simulink model "Conveyer_Belt_System"  (R2023a)
settings: Solver=VariableStepAuto  StartTime=0.0  StopTime=50  RelTol=1e-3
values from neighbouring files (symbols this model uses):
  Kb = 23e-3    (= 0.023)    [UpgradedConveyorBeltParameters.m]
  Kt = 23e-3    (= 0.023)    [UpgradedConveyorBeltParameters.m]
  L = 0.1    [UpgradedConveyorBeltParameters.m]
  R = 0.71    [UpgradedConveyorBeltParameters.m]
undefined symbols (not defined in the file or in its folder): J, Kd
libraries: SignalEditorBlockLib x4, slpidlib x1
settings Model: Creator=M3tal  LastModifiedBy=M3tal
settings ConfigComp: PLC_TargetIDE=generic  PLC_MultiTBSigbuilderTimeRange=off  PLC_FoldFBCallOutputVar=off  PLC_RemoveUnusedSSMethodCallArguments=off  PLC_UseCallOutputArgSyntax=off  PLC_EnableUnsignedAndDoubleTypes=off  PLC_EnableUDTSplitting=off  PLC_MaxFieldsInUDT=500  PLC_InlineEnumCastFunction=off

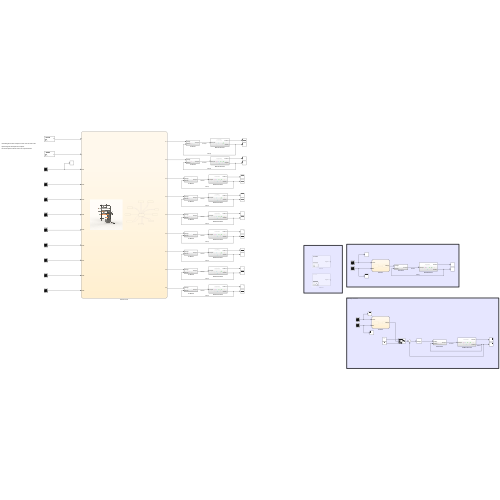
[thumbnail: Simulink's stored preview of the top-level diagram]
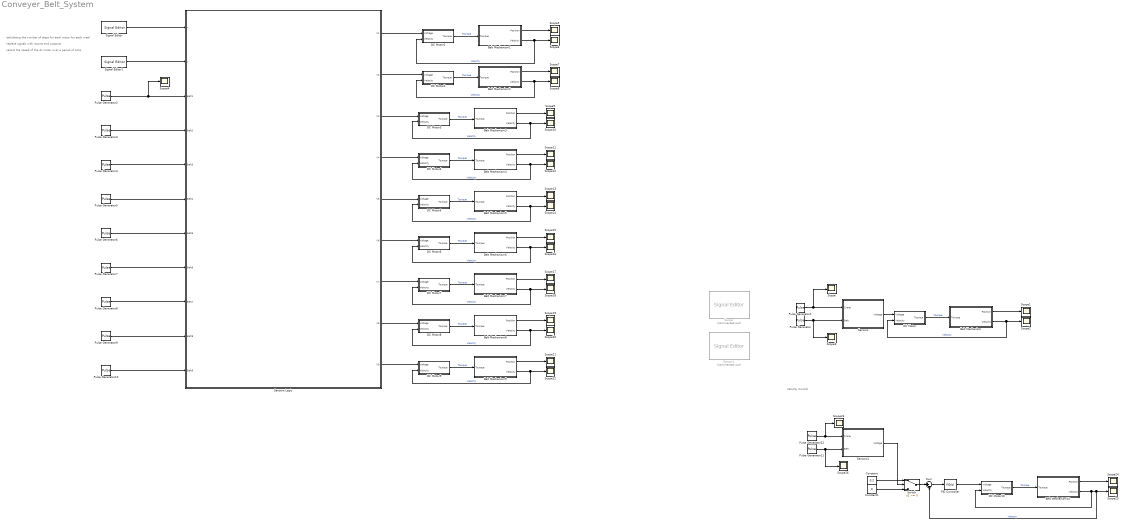
== system Conveyer_Belt_System ==
  note: -record the speed of the dc motor over a period of time
  note: -replace signals with inports and outports
  note: -caluclating the number of steps for each motor for each meal
  note: Velocity Control
  Belt Mechanism : Subsystem
  Belt Mechanism1 : Subsystem
  Belt Mechanism10 : Subsystem
  Belt Mechanism2 : Subsystem
  Belt Mechanism3 : Subsystem
  Belt Mechanism4 : Subsystem
  Belt Mechanism5 : Subsystem
  Belt Mechanism6 : Subsystem
  Belt Mechanism7 : Subsystem
  Belt Mechanism8 : Subsystem
  Belt Mechanism9 : Subsystem
  Constant : Constant  Value=0.2
  Constant1 : Constant  Value=0
  DC Motor : Subsystem
  DC Motor1 : Subsystem
  DC Motor10 : Subsystem
  DC Motor2 : Subsystem
  DC Motor3 : Subsystem
  DC Motor4 : Subsystem
  DC Motor5 : Subsystem
  DC Motor6 : Subsystem
  DC Motor7 : Subsystem
  DC Motor8 : Subsystem
  DC Motor9 : Subsystem
  PID Controller : slpidlib/PID Controller  Controller=PID  Form=Parallel  TimeDomain=Continuous-time  UseExternalTs=off  SampleTime=-1  IntegratorMethod=Forward Euler  FilterMethod=Forward Euler  ControllerParametersSource=internal  P=62.3819569355445  I=32.9771532942244  UseKiTs=off  D=11.2137291947193  N=1.39512955862012  UseFilter=on  TunerSelectOption=Transfer Function Based (PID Tuner App)  InitialConditionSource=internal  InitialConditionForIntegrator=0  InitialConditionForFilter=0  DifferentiatorICPrevScaledInput=0  ExternalReset=none  TrackingMode=off  Kt=1  LimitOutput=off  SatLimitsSource=internal  UpperSaturationLimit=inf  LowerSaturationLimit=-inf  LinearizeAsGain=on  AntiWindupMode=none  Kb=1  LimitIntegrator=off  UpperIntegratorSaturationLimit=inf  LowerIntegratorSaturationLimit=-inf  POutMin=[]  POutMax=[]  IOutMin=[]  IOutMax=[]  DOutMin=[]  DOutMax=[]  NOutMin=[]  NOutMax=[]  SumOutMin=[]  SumOutMax=[]  SaturationOutMin=[]  SaturationOutMax=[]  PParamMin=[]  PParamMax=[]  IParamMin=[]  IParamMax=[]  DParamMin=[]  DParamMax=[]  NParamMin=[]  NParamMax=[]  KbParamMin=[]  KbParamMax=[]  KtParamMin=[]  KtParamMax=[]  KbOutMin=[]  KbOutMax=[]  KtOutMin=[]  KtOutMax=[]  IntegratorOutMin=[]  IntegratorOutMax=[]  FilterOutMin=[]  FilterOutMax=[]  SumI1OutMin=[]  SumI1OutMax=[]  SumI2OutMin=[]  SumI2OutMax=[]  SumI3OutMin=[]  SumI3OutMax=[]  SumI4OutMin=[]  SumI4OutMax=[]  SumDOutMin=[]  SumDOutMax=[]  DifferentiatorOutMin=[]  DifferentiatorOutMax=[]  FilterDiffOutCoefMin=[]  FilterDiffOutCoefMax=[]  ReciprocalOutMin=[]  ReciprocalOutMax=[]  SumDenOutMin=[]  SumDenOutMax=[]  SumNumOutMin=[]  SumNumOutMax=[]  DivideOutMin=[]  DivideOutMax=[]  UdiffTsProdOutMin=[]  UdiffTsProdOutMax=[]  NTsProdOutMin=[]  NTsProdOutMax=[]  UintegralTsProdOutMin=[]  UintegralTsProdOutMax=[]  UngainTsProdOutMin=[]  UngainTsProdOutMax=[]  ClampingZeroOutDataTypeStr=Inherit: Inherit via back propagation  ClampingZeroOutMin=[]  ClampingZeroOutMax=[]  FilterDenConstantOutDataTypeStr=Inherit: Inherit via back propagation  FilterDenConstantOutMin=[]  FilterDenConstantOutMax=[]  PCopyOutDataTypeStr=Inherit: Inherit via back propagation  PCopyOutMin=[]  PCopyOutMax=[]  NCopyOutDataTypeStr=Inherit: Inherit via back propagation  NCopyOutMin=[]  NCopyOutMax=[]  IntegratorContinuousStateAttributes=''  IntegratorStateMustResolveToSignalObject=off  IntegratorRTWStateStorageClass=Auto  FilterContinuousStateAttributes=''  FilterStateMustResolveToSignalObject=off  FilterRTWStateStorageClass=Auto  ParallelPVariant=InternalParameters  IdealPVariant=Disabled  IVariant=InternalParameters  DVariant=InternalParameters  IntegratorVariant=Continuous  SatVariant=Disabled  AWVariant=Passthrough  PCopyVariant=Disabled  TRVariant=Disabled  FdbkBlocksVariant=Forward  IdealPFdbkVariant=Disabled  SatFdbkVariant=Disabled  DerivativeFilterVariant=ContFilter  NVariant=InternalParameters  NCopyVariant=Disabled  FilterICVariant=InternalICsFilter  IntegratorICVariant=InternalICs  ExternalResetVariant=Disabled  TRSumVariant=Passthrough  SumFdbkVariant=Disabled  SumVariant=Sum_PID  TsampFilterVariant=InternalTs  TsampNgainVariant=Passthrough  TsampIntegralVariant=Disabled_SignalSpec  ExternalSaturationOutDataTypeStr=Inherit: Same as second input
  Pulse Generator : DiscretePulseGenerator  PulseType=Time based  Period=40  PhaseDelay=20
  Pulse Generator1 : DiscretePulseGenerator  PulseType=Time based  Period=50  PhaseDelay=5
  Pulse Generator{3..10} (8 alike) : DiscretePulseGenerator  PulseType=Time based  Amplitude=0  Period=50  PhaseDelay=5
  Pulse Generator11 : DiscretePulseGenerator  PulseType=Time based  Period=40  PhaseDelay=20
  Pulse Generator12 : DiscretePulseGenerator  PulseType=Time based  Period=50  PhaseDelay=5
  Pulse Generator2 : DiscretePulseGenerator  PulseType=Time based  Period=50  PulseWidth=50  PhaseDelay=25
  Scope{,1..26} (27 alike) : Scope
  Sensor : SignalEditorBlockLib/Signal Editor  Commented=on  FileName=Crane_Sensor.mat  ActiveScenario=Scenario  ActiveSignal=Crane signal  IsBus=off  OutputBusObjectStr=Bus: BusObject  SampleTime=0  Interpolate=off  ZeroCross=off  OutputAfterFinalValue=Setting to zero  Unit=inherit  PreserveSignalName=on  ApplySigPropsToAllScenarios=on
  Sensor1 : SignalEditorBlockLib/Signal Editor  Commented=on  FileName=Belt_Sensor.mat  ActiveScenario=Scenario  ActiveSignal=Belt Signal  IsBus=off  OutputBusObjectStr=Bus: BusObject  SampleTime=0  Interpolate=off  ZeroCross=off  OutputAfterFinalValue=Setting to zero  Unit=inherit  PreserveSignalName=on  ApplySigPropsToAllScenarios=on
  Sensors : Stateflow chart  TreatAsAtomicUnit=on
  Sensors Logic : Stateflow chart  TreatAsAtomicUnit=on
      settings: PortSchema="{\"entries\":[{\"content\":{\"sides\":[{\"content\":{\"connectorIds\":[\"In10\",\"In11\",\"In1\",\"In2\",\"In3\",\"In4\",\"In5\",\"In6\",\"In7\",\"In8\",\"In9\"]},\"type\":\"ConnectorPlacement.EquallySpacedRectSide\",\"uuid\":\"dd9ce701-3689-4654-9b21-5529dab0541a\"},{\"content\":{\"connectorIds\":[\"Out1\",\"Out2\",\"Out3\",\"Out4\",\"Out5\",\"Out6\",\"Out7\",\"Out8\",\"Out9\"],\"side\":\"RIGHT\"},\"type\":\"ConnectorPlacement.EquallySpacedRectSide\",\"uuid\":\"ff8f0f67-846c-4703-aeda-d87216d47c92\"},{\"content\":{\"side\":\"TOP\"},\"type\":\"ConnectorPlacement.EquallySpacedRectSide\",\"uuid\":\"ae968bb7-da0f-44fd-802b-06f57922bbce\"}]},\"type\":\"ConnectorPlacement.EquallySpacedConnector\",\"uuid\":\"820653e5-881f-4b8b-9810-894dc5dde637\"}],\"packageUris\":[\"http://schema.mathworks.com/mf0/Connector/R2020b\"],\"version\":\"1.0\"}"
  Sensors1 : Stateflow chart  TreatAsAtomicUnit=on
  Signal Editor : SignalEditorBlockLib/Signal Editor  FileName=X_Position.mat  ActiveScenario=Scenario  ActiveSignal=X  IsBus=off  OutputBusObjectStr=Bus: BusObject  SampleTime=0  Interpolate=off  ZeroCross=off  OutputAfterFinalValue=Setting to zero  Unit=inherit  PreserveSignalName=on  ApplySigPropsToAllScenarios=on
  Signal Editor1 : SignalEditorBlockLib/Signal Editor  FileName=Y_Position.mat  ActiveScenario=Scenario  ActiveSignal=Y  IsBus=off  OutputBusObjectStr=Bus: BusObject  SampleTime=0  Interpolate=off  ZeroCross=off  OutputAfterFinalValue=Setting to zero  Unit=inherit  PreserveSignalName=on  ApplySigPropsToAllScenarios=on
  Sum : Sum  Inputs=|+-
  Switch : Switch  Criteria=u2 ~= 0  Threshold=1  SaturateOnIntegerOverflow=off  InputSameDT=off
  wires:
  Belt Mechanism/1(Position) -> Scope1/1
  DC Motor/1(Tourque) -> Belt Mechanism/1(Tourque)  "Tourque"
  Belt Mechanism/2(Velocity) -> Scope2/1, DC Motor/2(Velocity)  "Velocity"
  Pulse Generator/1 -> Scope3/1, Sensors/2(Belt)
  Pulse Generator1/1 -> Scope/1, Sensors/1(Crane)
  Pulse Generator2/1 -> Scope4/1, Sensors Logic/1(Belt1)
  Pulse Generator3/1 -> Sensors Logic/2(Belt2)
  Pulse Generator4/1 -> Sensors Logic/3(Belt3)
  Pulse Generator5/1 -> Sensors Logic/4(Belt4)
  Pulse Generator6/1 -> Sensors Logic/5(Belt5)
  Pulse Generator7/1 -> Sensors Logic/6(Belt6)
  Pulse Generator8/1 -> Sensors Logic/7(Belt7)
  Pulse Generator9/1 -> Sensors Logic/8(Belt8)
  Pulse Generator10/1 -> Sensors Logic/9(Belt9)
  Signal Editor1/1 -> Sensors Logic/11(y)
  Signal Editor/1 -> Sensors Logic/10(x)
  Belt Mechanism1/2(Velocity) -> Scope6/1, DC Motor1/2(Velocity)  "Velocity"
  DC Motor1/1(Tourque) -> Belt Mechanism1/1(Tourque)  "Tourque"
  Belt Mechanism1/1(Position) -> Scope5/1
  Belt Mechanism2/1(Position) -> Scope7/1
  DC Motor2/1(Tourque) -> Belt Mechanism2/1(Tourque)  "Tourque"
  Belt Mechanism2/2(Velocity) -> Scope8/1, DC Motor2/2(Velocity)  "Velocity"
  Belt Mechanism3/1(Position) -> Scope9/1
  DC Motor3/1(Tourque) -> Belt Mechanism3/1(Tourque)  "Tourque"
  Belt Mechanism3/2(Velocity) -> Scope10/1, DC Motor3/2(Velocity)  "Velocity"
  Belt Mechanism4/1(Position) -> Scope11/1
  DC Motor4/1(Tourque) -> Belt Mechanism4/1(Tourque)  "Tourque"
  Belt Mechanism4/2(Velocity) -> Scope12/1, DC Motor4/2(Velocity)  "Velocity"
  Belt Mechanism5/1(Position) -> Scope13/1
  DC Motor5/1(Tourque) -> Belt Mechanism5/1(Tourque)  "Tourque"
  Belt Mechanism5/2(Velocity) -> Scope14/1, DC Motor5/2(Velocity)  "Velocity"
  Belt Mechanism6/1(Position) -> Scope15/1
  DC Motor6/1(Tourque) -> Belt Mechanism6/1(Tourque)  "Tourque"
  Belt Mechanism6/2(Velocity) -> Scope16/1, DC Motor6/2(Velocity)  "Velocity"
  Belt Mechanism7/1(Position) -> Scope17/1
  DC Motor7/1(Tourque) -> Belt Mechanism7/1(Tourque)  "Tourque"
  Belt Mechanism7/2(Velocity) -> Scope18/1, DC Motor7/2(Velocity)  "Velocity"
  Belt Mechanism8/1(Position) -> Scope19/1
  DC Motor8/1(Tourque) -> Belt Mechanism8/1(Tourque)  "Tourque"
  Belt Mechanism8/2(Velocity) -> Scope20/1, DC Motor8/2(Velocity)  "Velocity"
  Belt Mechanism9/1(Position) -> Scope21/1
  DC Motor9/1(Tourque) -> Belt Mechanism9/1(Tourque)  "Tourque"
  Belt Mechanism9/2(Velocity) -> Scope22/1, DC Motor9/2(Velocity)  "Velocity"
  Sensors Logic/1(V1) -> DC Motor1/1(Voltage)
  Sensors Logic/2(V2) -> DC Motor2/1(Voltage)
  Sensors Logic/3(V3) -> DC Motor3/1(Voltage)
  Sensors Logic/4(V4) -> DC Motor4/1(Voltage)
  Sensors Logic/5(V5) -> DC Motor5/1(Voltage)
  Sensors Logic/6(V6) -> DC Motor6/1(Voltage)
  Sensors Logic/7(V7) -> DC Motor7/1(Voltage)
  Sensors Logic/8(V8) -> DC Motor8/1(Voltage)
  Sensors Logic/9(V9) -> DC Motor9/1(Voltage)
  Sensors/1(Voltage) -> DC Motor/1(Voltage)
  Constant1/1 -> Switch/3
  Sum/1 -> PID Controller/1
  Belt Mechanism10/1(Position) -> Scope24/1
  Pulse Generator11/1 -> Scope26/1, Sensors1/2(Belt)
  DC Motor10/1(Tourque) -> Belt Mechanism10/1(Tourque)  "Tourque"
  Sensors1/1(Voltage) -> Switch/2
  Constant/1 -> Switch/1
  Pulse Generator12/1 -> Scope23/1, Sensors1/1(Crane)
  Belt Mechanism10/2(Velocity) -> DC Motor10/2(Velocity), Sum/2, Scope25/1  "Velocity"
  PID Controller/1 -> DC Motor10/1(Voltage)
  Switch/1 -> Sum/1

== system Conveyer_Belt_System/Belt Mechanism ==
  note: Note: The term $K \frac{d\theta}{dt}$ ​ represents a damping torque that is proportional to the angular velocity
  note: $\frac{d^2\theta}{dt^2} = \frac{1}{J} \left(T - K \frac{d\theta}{dt}\right)$
      | belt mechanism equaition based on newton seconed law for rotational motion
  Tourque : Inport
  Gain1 : Gain  Gain=1/J
  Integrator2 : Integrator
  Integrator3 : Integrator
  Subtract : Sum  Inputs=+-
  damping coefficient : Gain  Gain=Kd
  Position : Outport
  Velocity : Outport  Port=2
  wires:
  Integrator2/1 -> damping coefficient/1, Velocity/1, Integrator3/1  "Velocity"
  Tourque/1 -> Subtract/1
  Subtract/1 -> Gain1/1
  Integrator3/1 -> Position/1  "Position"
  damping coefficient/1 -> Subtract/2
  Gain1/1 -> Integrator2/1  "theta_dot_dot"

== system Conveyer_Belt_System/Belt Mechanism1 ==
  note: Note: The term $K \frac{d\theta}{dt}$ ​ represents a damping torque that is proportional to the angular velocity
  note: $\frac{d^2\theta}{dt^2} = \frac{1}{J} \left(T - K \frac{d\theta}{dt}\right)$
      | belt mechanism equaition based on newton seconed law for rotational motion
  Tourque : Inport
  Gain1 : Gain  Gain=1/J
  Integrator2 : Integrator
  Integrator3 : Integrator
  Subtract : Sum  Inputs=+-
  damping coefficient : Gain  Gain=Kd
  Position : Outport
  Velocity : Outport  Port=2
  wires:
  Integrator2/1 -> damping coefficient/1, Velocity/1, Integrator3/1  "Velocity"
  Tourque/1 -> Subtract/1
  Subtract/1 -> Gain1/1
  Integrator3/1 -> Position/1  "Position"
  damping coefficient/1 -> Subtract/2
  Gain1/1 -> Integrator2/1  "theta_dot_dot"

== system Conveyer_Belt_System/Belt Mechanism10 ==
  note: Note: The term $K \frac{d\theta}{dt}$ ​ represents a damping torque that is proportional to the angular velocity
  note: $\frac{d^2\theta}{dt^2} = \frac{1}{J} \left(T - K \frac{d\theta}{dt}\right)$
      | belt mechanism equaition based on newton seconed law for rotational motion
  Tourque : Inport
  Gain1 : Gain  Gain=1/J
  Integrator2 : Integrator
  Integrator3 : Integrator
  Subtract : Sum  Inputs=+-
  damping coefficient : Gain  Gain=Kd
  Position : Outport
  Velocity : Outport  Port=2
  wires:
  Integrator2/1 -> damping coefficient/1, Velocity/1, Integrator3/1  "Velocity"
  Tourque/1 -> Subtract/1
  Subtract/1 -> Gain1/1
  Integrator3/1 -> Position/1  "Position"
  damping coefficient/1 -> Subtract/2
  Gain1/1 -> Integrator2/1  "theta_dot_dot"

== system Conveyer_Belt_System/Belt Mechanism2 ==
  note: Note: The term $K \frac{d\theta}{dt}$ ​ represents a damping torque that is proportional to the angular velocity
  note: $\frac{d^2\theta}{dt^2} = \frac{1}{J} \left(T - K \frac{d\theta}{dt}\right)$
      | belt mechanism equaition based on newton seconed law for rotational motion
  Tourque : Inport
  Gain1 : Gain  Gain=1/J
  Integrator2 : Integrator
  Integrator3 : Integrator
  Subtract : Sum  Inputs=+-
  damping coefficient : Gain  Gain=Kd
  Position : Outport
  Velocity : Outport  Port=2
  wires:
  Integrator2/1 -> damping coefficient/1, Velocity/1, Integrator3/1  "Velocity"
  Tourque/1 -> Subtract/1
  Subtract/1 -> Gain1/1
  Integrator3/1 -> Position/1  "Position"
  damping coefficient/1 -> Subtract/2
  Gain1/1 -> Integrator2/1  "theta_dot_dot"

== system Conveyer_Belt_System/Belt Mechanism3 ==
  note: Note: The term $K \frac{d\theta}{dt}$ ​ represents a damping torque that is proportional to the angular velocity
  note: $\frac{d^2\theta}{dt^2} = \frac{1}{J} \left(T - K \frac{d\theta}{dt}\right)$
      | belt mechanism equaition based on newton seconed law for rotational motion
  Tourque : Inport
  Gain1 : Gain  Gain=1/J
  Integrator2 : Integrator
  Integrator3 : Integrator
  Subtract : Sum  Inputs=+-
  damping coefficient : Gain  Gain=Kd
  Position : Outport
  Velocity : Outport  Port=2
  wires:
  Integrator2/1 -> damping coefficient/1, Velocity/1, Integrator3/1  "Velocity"
  Tourque/1 -> Subtract/1
  Subtract/1 -> Gain1/1
  Integrator3/1 -> Position/1  "Position"
  damping coefficient/1 -> Subtract/2
  Gain1/1 -> Integrator2/1  "theta_dot_dot"

== system Conveyer_Belt_System/Belt Mechanism4 ==
  note: Note: The term $K \frac{d\theta}{dt}$ ​ represents a damping torque that is proportional to the angular velocity
  note: $\frac{d^2\theta}{dt^2} = \frac{1}{J} \left(T - K \frac{d\theta}{dt}\right)$
      | belt mechanism equaition based on newton seconed law for rotational motion
  Tourque : Inport
  Gain1 : Gain  Gain=1/J
  Integrator2 : Integrator
  Integrator3 : Integrator
  Subtract : Sum  Inputs=+-
  damping coefficient : Gain  Gain=Kd
  Position : Outport
  Velocity : Outport  Port=2
  wires:
  Integrator2/1 -> damping coefficient/1, Velocity/1, Integrator3/1  "Velocity"
  Tourque/1 -> Subtract/1
  Subtract/1 -> Gain1/1
  Integrator3/1 -> Position/1  "Position"
  damping coefficient/1 -> Subtract/2
  Gain1/1 -> Integrator2/1  "theta_dot_dot"

== system Conveyer_Belt_System/Belt Mechanism5 ==
  note: Note: The term $K \frac{d\theta}{dt}$ ​ represents a damping torque that is proportional to the angular velocity
  note: $\frac{d^2\theta}{dt^2} = \frac{1}{J} \left(T - K \frac{d\theta}{dt}\right)$
      | belt mechanism equaition based on newton seconed law for rotational motion
  Tourque : Inport
  Gain1 : Gain  Gain=1/J
  Integrator2 : Integrator
  Integrator3 : Integrator
  Subtract : Sum  Inputs=+-
  damping coefficient : Gain  Gain=Kd
  Position : Outport
  Velocity : Outport  Port=2
  wires:
  Integrator2/1 -> damping coefficient/1, Velocity/1, Integrator3/1  "Velocity"
  Tourque/1 -> Subtract/1
  Subtract/1 -> Gain1/1
  Integrator3/1 -> Position/1  "Position"
  damping coefficient/1 -> Subtract/2
  Gain1/1 -> Integrator2/1  "theta_dot_dot"

== system Conveyer_Belt_System/Belt Mechanism6 ==
  note: Note: The term $K \frac{d\theta}{dt}$ ​ represents a damping torque that is proportional to the angular velocity
  note: $\frac{d^2\theta}{dt^2} = \frac{1}{J} \left(T - K \frac{d\theta}{dt}\right)$
      | belt mechanism equaition based on newton seconed law for rotational motion
  Tourque : Inport
  Gain1 : Gain  Gain=1/J
  Integrator2 : Integrator
  Integrator3 : Integrator
  Subtract : Sum  Inputs=+-
  damping coefficient : Gain  Gain=Kd
  Position : Outport
  Velocity : Outport  Port=2
  wires:
  Integrator2/1 -> damping coefficient/1, Velocity/1, Integrator3/1  "Velocity"
  Tourque/1 -> Subtract/1
  Subtract/1 -> Gain1/1
  Integrator3/1 -> Position/1  "Position"
  damping coefficient/1 -> Subtract/2
  Gain1/1 -> Integrator2/1  "theta_dot_dot"

== system Conveyer_Belt_System/Belt Mechanism7 ==
  note: Note: The term $K \frac{d\theta}{dt}$ ​ represents a damping torque that is proportional to the angular velocity
  note: $\frac{d^2\theta}{dt^2} = \frac{1}{J} \left(T - K \frac{d\theta}{dt}\right)$
      | belt mechanism equaition based on newton seconed law for rotational motion
  Tourque : Inport
  Gain1 : Gain  Gain=1/J
  Integrator2 : Integrator
  Integrator3 : Integrator
  Subtract : Sum  Inputs=+-
  damping coefficient : Gain  Gain=Kd
  Position : Outport
  Velocity : Outport  Port=2
  wires:
  Integrator2/1 -> damping coefficient/1, Velocity/1, Integrator3/1  "Velocity"
  Tourque/1 -> Subtract/1
  Subtract/1 -> Gain1/1
  Integrator3/1 -> Position/1  "Position"
  damping coefficient/1 -> Subtract/2
  Gain1/1 -> Integrator2/1  "theta_dot_dot"

== system Conveyer_Belt_System/Belt Mechanism8 ==
  note: Note: The term $K \frac{d\theta}{dt}$ ​ represents a damping torque that is proportional to the angular velocity
  note: $\frac{d^2\theta}{dt^2} = \frac{1}{J} \left(T - K \frac{d\theta}{dt}\right)$
      | belt mechanism equaition based on newton seconed law for rotational motion
  Tourque : Inport
  Gain1 : Gain  Gain=1/J
  Integrator2 : Integrator
  Integrator3 : Integrator
  Subtract : Sum  Inputs=+-
  damping coefficient : Gain  Gain=Kd
  Position : Outport
  Velocity : Outport  Port=2
  wires:
  Integrator2/1 -> damping coefficient/1, Velocity/1, Integrator3/1  "Velocity"
  Tourque/1 -> Subtract/1
  Subtract/1 -> Gain1/1
  Integrator3/1 -> Position/1  "Position"
  damping coefficient/1 -> Subtract/2
  Gain1/1 -> Integrator2/1  "theta_dot_dot"

== system Conveyer_Belt_System/Belt Mechanism9 ==
  note: Note: The term $K \frac{d\theta}{dt}$ ​ represents a damping torque that is proportional to the angular velocity
  note: $\frac{d^2\theta}{dt^2} = \frac{1}{J} \left(T - K \frac{d\theta}{dt}\right)$
      | belt mechanism equaition based on newton seconed law for rotational motion
  Tourque : Inport
  Gain1 : Gain  Gain=1/J
  Integrator2 : Integrator
  Integrator3 : Integrator
  Subtract : Sum  Inputs=+-
  damping coefficient : Gain  Gain=Kd
  Position : Outport
  Velocity : Outport  Port=2
  wires:
  Integrator2/1 -> damping coefficient/1, Velocity/1, Integrator3/1  "Velocity"
  Tourque/1 -> Subtract/1
  Subtract/1 -> Gain1/1
  Integrator3/1 -> Position/1  "Position"
  damping coefficient/1 -> Subtract/2
  Gain1/1 -> Integrator2/1  "theta_dot_dot"

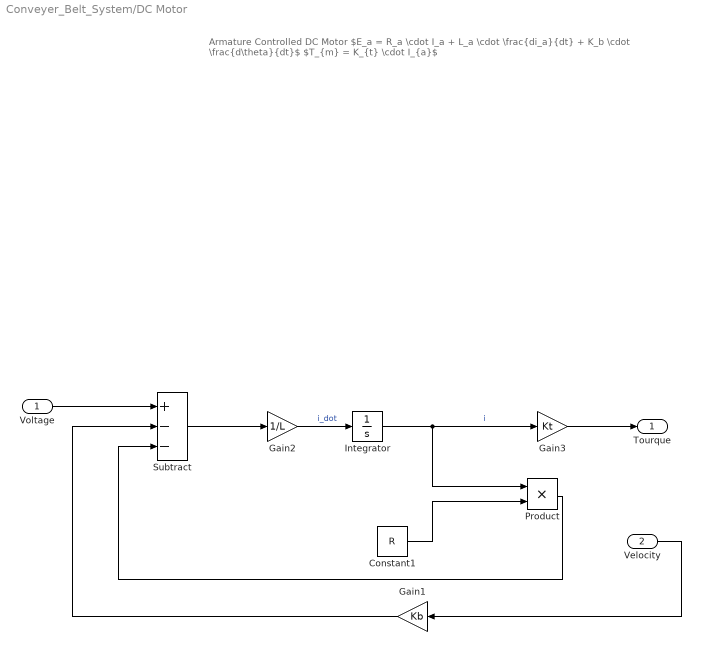
== system Conveyer_Belt_System/DC Motor ==
  note: Armature Controlled DC Motor
      |
      | $E_a = R_a \cdot I_a + L_a \cdot \frac{di_a}{dt} + K_b \cdot \frac{d\theta}{dt}$
      | $T_{m} = K_{t} \cdot I_{a}$
  Voltage : Inport
  Velocity : Inport  Port=2
  Constant1 : Constant  Value=R
  Gain1 : Gain  Gain=Kb
  Gain2 : Gain  Gain=1/L
  Gain3 : Gain  Gain=Kt
  Integrator : Integrator
  Product : Product
  Subtract : Sum  Inputs=+--
  Tourque : Outport
  wires:
  Voltage/1 -> Subtract/1
  Integrator/1 -> Product/1, Gain3/1  "i"
  Gain3/1 -> Tourque/1
  Gain1/1 -> Subtract/2
  Velocity/1 -> Gain1/1
  Constant1/1 -> Product/2
  Product/1 -> Subtract/3
  Gain2/1 -> Integrator/1  "i_dot"
  Subtract/1 -> Gain2/1

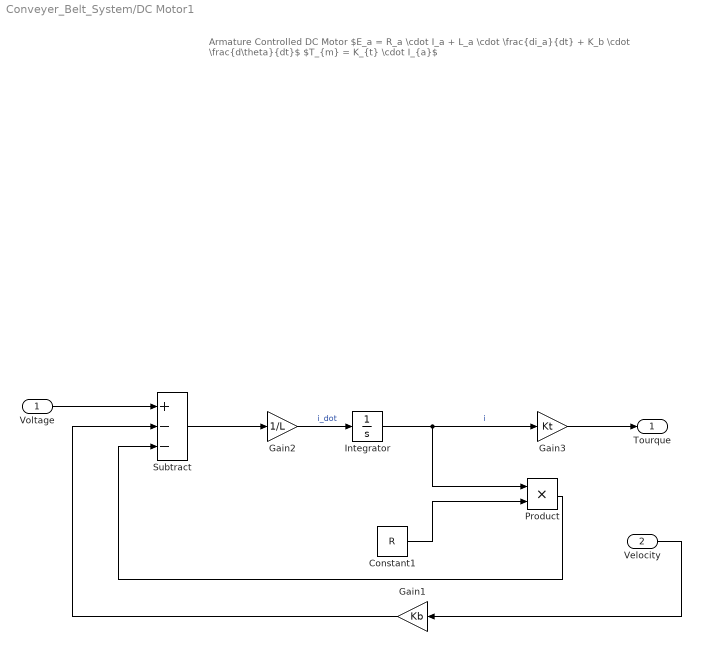
== system Conveyer_Belt_System/DC Motor1 ==
  note: Armature Controlled DC Motor
      |
      | $E_a = R_a \cdot I_a + L_a \cdot \frac{di_a}{dt} + K_b \cdot \frac{d\theta}{dt}$
      | $T_{m} = K_{t} \cdot I_{a}$
  Voltage : Inport
  Velocity : Inport  Port=2
  Constant1 : Constant  Value=R
  Gain1 : Gain  Gain=Kb
  Gain2 : Gain  Gain=1/L
  Gain3 : Gain  Gain=Kt
  Integrator : Integrator
  Product : Product
  Subtract : Sum  Inputs=+--
  Tourque : Outport
  wires:
  Voltage/1 -> Subtract/1
  Integrator/1 -> Product/1, Gain3/1  "i"
  Gain3/1 -> Tourque/1
  Gain1/1 -> Subtract/2
  Velocity/1 -> Gain1/1
  Constant1/1 -> Product/2
  Product/1 -> Subtract/3
  Gain2/1 -> Integrator/1  "i_dot"
  Subtract/1 -> Gain2/1

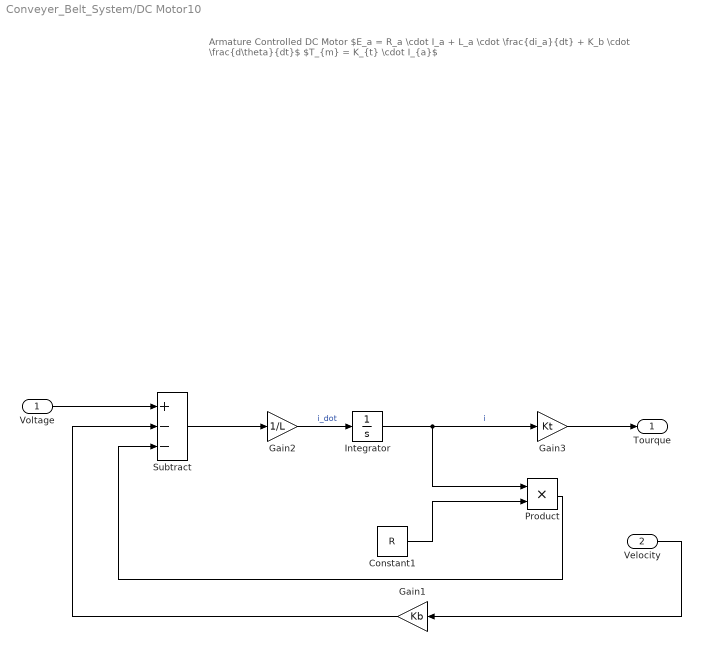
== system Conveyer_Belt_System/DC Motor10 ==
  note: Armature Controlled DC Motor
      |
      | $E_a = R_a \cdot I_a + L_a \cdot \frac{di_a}{dt} + K_b \cdot \frac{d\theta}{dt}$
      | $T_{m} = K_{t} \cdot I_{a}$
  Voltage : Inport
  Velocity : Inport  Port=2
  Constant1 : Constant  Value=R
  Gain1 : Gain  Gain=Kb
  Gain2 : Gain  Gain=1/L
  Gain3 : Gain  Gain=Kt
  Integrator : Integrator
  Product : Product
  Subtract : Sum  Inputs=+--
  Tourque : Outport
  wires:
  Voltage/1 -> Subtract/1
  Integrator/1 -> Product/1, Gain3/1  "i"
  Gain3/1 -> Tourque/1
  Gain1/1 -> Subtract/2
  Velocity/1 -> Gain1/1
  Constant1/1 -> Product/2
  Product/1 -> Subtract/3
  Gain2/1 -> Integrator/1  "i_dot"
  Subtract/1 -> Gain2/1

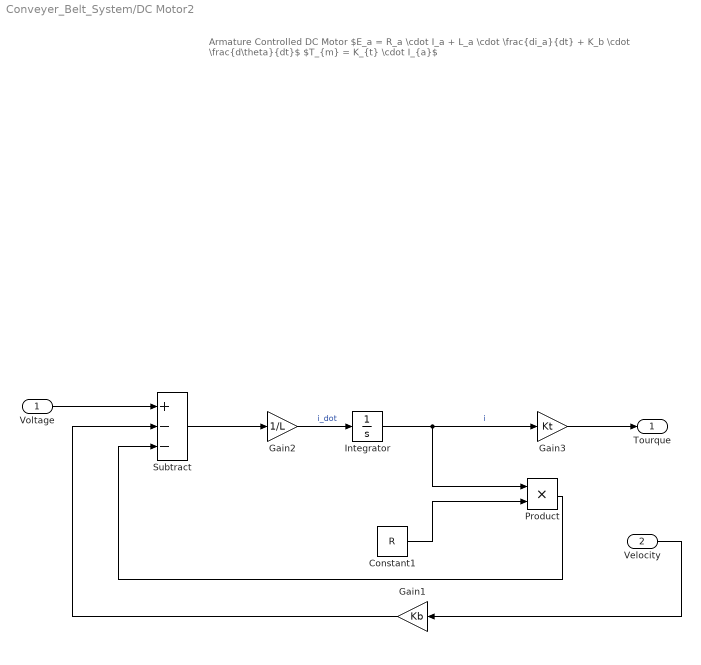
== system Conveyer_Belt_System/DC Motor2 ==
  note: Armature Controlled DC Motor
      |
      | $E_a = R_a \cdot I_a + L_a \cdot \frac{di_a}{dt} + K_b \cdot \frac{d\theta}{dt}$
      | $T_{m} = K_{t} \cdot I_{a}$
  Voltage : Inport
  Velocity : Inport  Port=2
  Constant1 : Constant  Value=R
  Gain1 : Gain  Gain=Kb
  Gain2 : Gain  Gain=1/L
  Gain3 : Gain  Gain=Kt
  Integrator : Integrator
  Product : Product
  Subtract : Sum  Inputs=+--
  Tourque : Outport
  wires:
  Voltage/1 -> Subtract/1
  Integrator/1 -> Product/1, Gain3/1  "i"
  Gain3/1 -> Tourque/1
  Gain1/1 -> Subtract/2
  Velocity/1 -> Gain1/1
  Constant1/1 -> Product/2
  Product/1 -> Subtract/3
  Gain2/1 -> Integrator/1  "i_dot"
  Subtract/1 -> Gain2/1

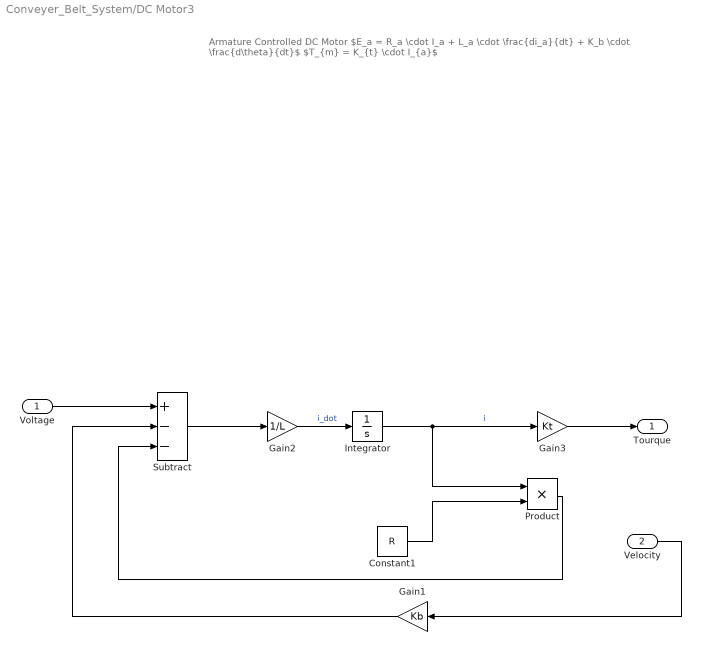
== system Conveyer_Belt_System/DC Motor3 ==
  note: Armature Controlled DC Motor
      |
      | $E_a = R_a \cdot I_a + L_a \cdot \frac{di_a}{dt} + K_b \cdot \frac{d\theta}{dt}$
      | $T_{m} = K_{t} \cdot I_{a}$
  Voltage : Inport
  Velocity : Inport  Port=2
  Constant1 : Constant  Value=R
  Gain1 : Gain  Gain=Kb
  Gain2 : Gain  Gain=1/L
  Gain3 : Gain  Gain=Kt
  Integrator : Integrator
  Product : Product
  Subtract : Sum  Inputs=+--
  Tourque : Outport
  wires:
  Voltage/1 -> Subtract/1
  Integrator/1 -> Product/1, Gain3/1  "i"
  Gain3/1 -> Tourque/1
  Gain1/1 -> Subtract/2
  Velocity/1 -> Gain1/1
  Constant1/1 -> Product/2
  Product/1 -> Subtract/3
  Gain2/1 -> Integrator/1  "i_dot"
  Subtract/1 -> Gain2/1

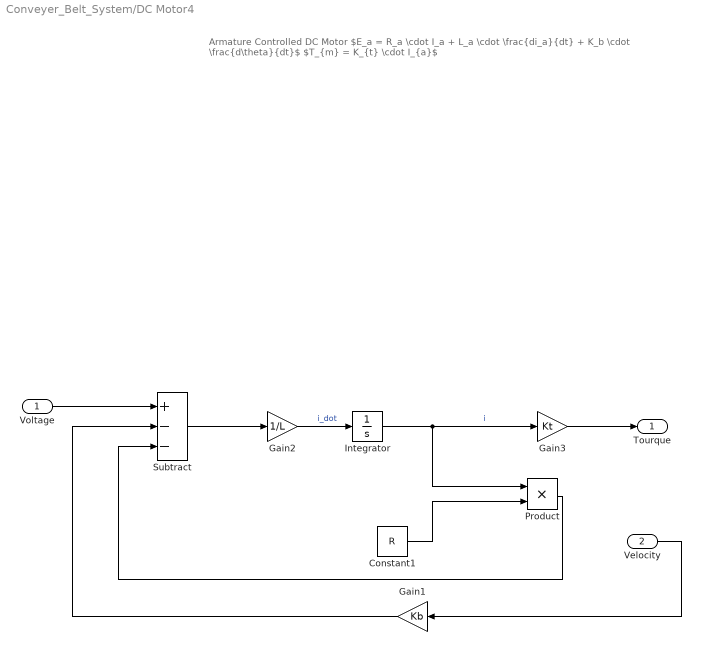
== system Conveyer_Belt_System/DC Motor4 ==
  note: Armature Controlled DC Motor
      |
      | $E_a = R_a \cdot I_a + L_a \cdot \frac{di_a}{dt} + K_b \cdot \frac{d\theta}{dt}$
      | $T_{m} = K_{t} \cdot I_{a}$
  Voltage : Inport
  Velocity : Inport  Port=2
  Constant1 : Constant  Value=R
  Gain1 : Gain  Gain=Kb
  Gain2 : Gain  Gain=1/L
  Gain3 : Gain  Gain=Kt
  Integrator : Integrator
  Product : Product
  Subtract : Sum  Inputs=+--
  Tourque : Outport
  wires:
  Voltage/1 -> Subtract/1
  Integrator/1 -> Product/1, Gain3/1  "i"
  Gain3/1 -> Tourque/1
  Gain1/1 -> Subtract/2
  Velocity/1 -> Gain1/1
  Constant1/1 -> Product/2
  Product/1 -> Subtract/3
  Gain2/1 -> Integrator/1  "i_dot"
  Subtract/1 -> Gain2/1

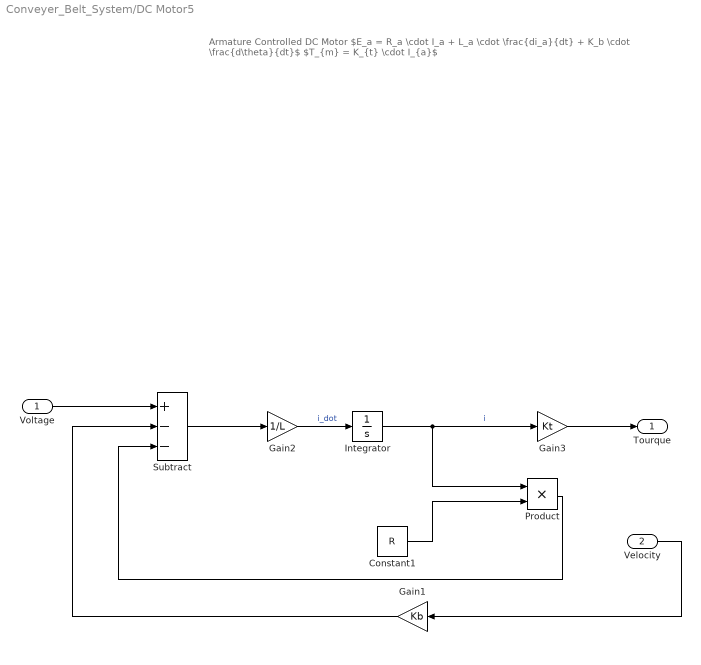
== system Conveyer_Belt_System/DC Motor5 ==
  note: Armature Controlled DC Motor
      |
      | $E_a = R_a \cdot I_a + L_a \cdot \frac{di_a}{dt} + K_b \cdot \frac{d\theta}{dt}$
      | $T_{m} = K_{t} \cdot I_{a}$
  Voltage : Inport
  Velocity : Inport  Port=2
  Constant1 : Constant  Value=R
  Gain1 : Gain  Gain=Kb
  Gain2 : Gain  Gain=1/L
  Gain3 : Gain  Gain=Kt
  Integrator : Integrator
  Product : Product
  Subtract : Sum  Inputs=+--
  Tourque : Outport
  wires:
  Voltage/1 -> Subtract/1
  Integrator/1 -> Product/1, Gain3/1  "i"
  Gain3/1 -> Tourque/1
  Gain1/1 -> Subtract/2
  Velocity/1 -> Gain1/1
  Constant1/1 -> Product/2
  Product/1 -> Subtract/3
  Gain2/1 -> Integrator/1  "i_dot"
  Subtract/1 -> Gain2/1

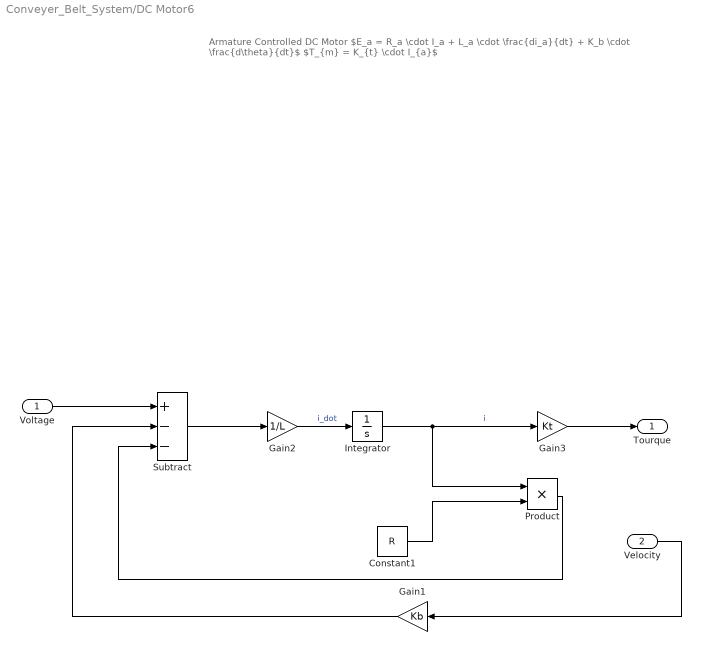
== system Conveyer_Belt_System/DC Motor6 ==
  note: Armature Controlled DC Motor
      |
      | $E_a = R_a \cdot I_a + L_a \cdot \frac{di_a}{dt} + K_b \cdot \frac{d\theta}{dt}$
      | $T_{m} = K_{t} \cdot I_{a}$
  Voltage : Inport
  Velocity : Inport  Port=2
  Constant1 : Constant  Value=R
  Gain1 : Gain  Gain=Kb
  Gain2 : Gain  Gain=1/L
  Gain3 : Gain  Gain=Kt
  Integrator : Integrator
  Product : Product
  Subtract : Sum  Inputs=+--
  Tourque : Outport
  wires:
  Voltage/1 -> Subtract/1
  Integrator/1 -> Product/1, Gain3/1  "i"
  Gain3/1 -> Tourque/1
  Gain1/1 -> Subtract/2
  Velocity/1 -> Gain1/1
  Constant1/1 -> Product/2
  Product/1 -> Subtract/3
  Gain2/1 -> Integrator/1  "i_dot"
  Subtract/1 -> Gain2/1

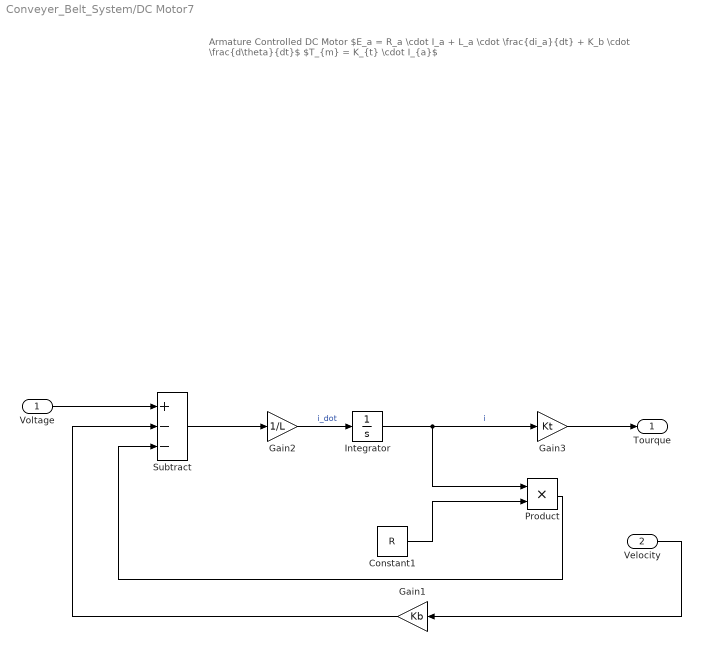
== system Conveyer_Belt_System/DC Motor7 ==
  note: Armature Controlled DC Motor
      |
      | $E_a = R_a \cdot I_a + L_a \cdot \frac{di_a}{dt} + K_b \cdot \frac{d\theta}{dt}$
      | $T_{m} = K_{t} \cdot I_{a}$
  Voltage : Inport
  Velocity : Inport  Port=2
  Constant1 : Constant  Value=R
  Gain1 : Gain  Gain=Kb
  Gain2 : Gain  Gain=1/L
  Gain3 : Gain  Gain=Kt
  Integrator : Integrator
  Product : Product
  Subtract : Sum  Inputs=+--
  Tourque : Outport
  wires:
  Voltage/1 -> Subtract/1
  Integrator/1 -> Product/1, Gain3/1  "i"
  Gain3/1 -> Tourque/1
  Gain1/1 -> Subtract/2
  Velocity/1 -> Gain1/1
  Constant1/1 -> Product/2
  Product/1 -> Subtract/3
  Gain2/1 -> Integrator/1  "i_dot"
  Subtract/1 -> Gain2/1

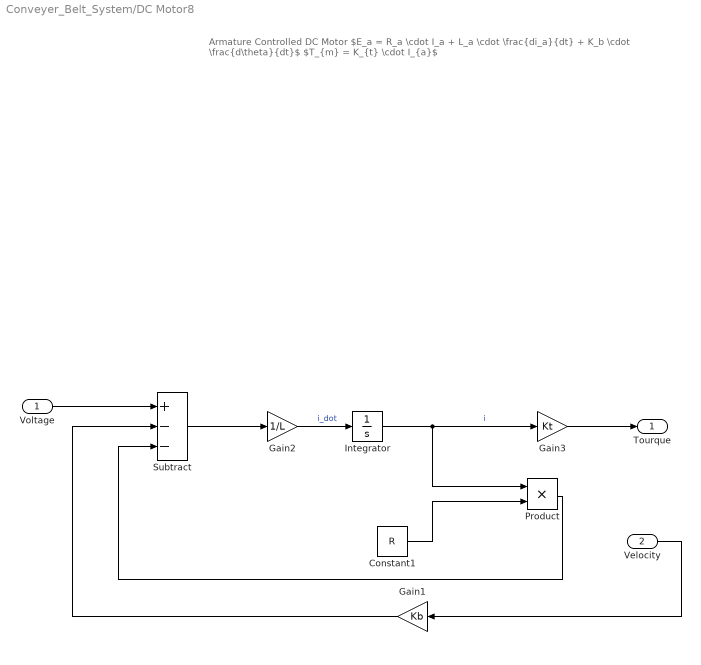
== system Conveyer_Belt_System/DC Motor8 ==
  note: Armature Controlled DC Motor
      |
      | $E_a = R_a \cdot I_a + L_a \cdot \frac{di_a}{dt} + K_b \cdot \frac{d\theta}{dt}$
      | $T_{m} = K_{t} \cdot I_{a}$
  Voltage : Inport
  Velocity : Inport  Port=2
  Constant1 : Constant  Value=R
  Gain1 : Gain  Gain=Kb
  Gain2 : Gain  Gain=1/L
  Gain3 : Gain  Gain=Kt
  Integrator : Integrator
  Product : Product
  Subtract : Sum  Inputs=+--
  Tourque : Outport
  wires:
  Voltage/1 -> Subtract/1
  Integrator/1 -> Product/1, Gain3/1  "i"
  Gain3/1 -> Tourque/1
  Gain1/1 -> Subtract/2
  Velocity/1 -> Gain1/1
  Constant1/1 -> Product/2
  Product/1 -> Subtract/3
  Gain2/1 -> Integrator/1  "i_dot"
  Subtract/1 -> Gain2/1

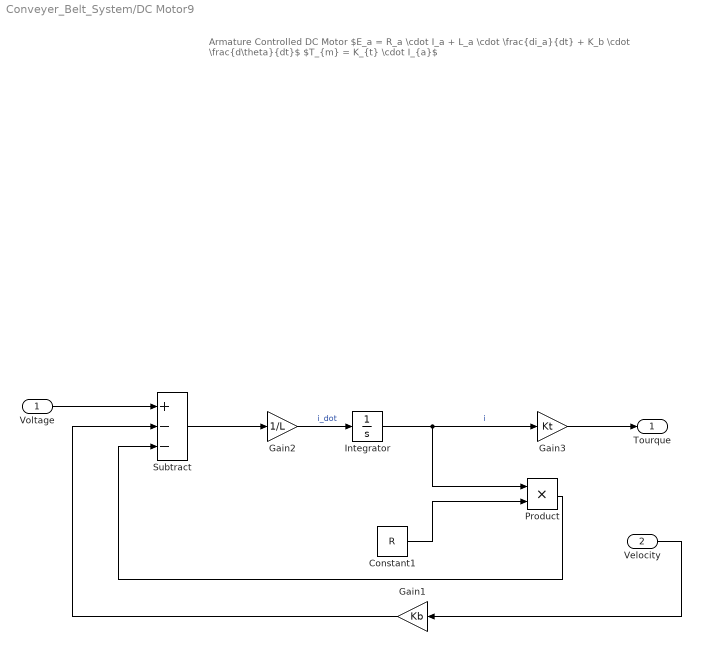
== system Conveyer_Belt_System/DC Motor9 ==
  note: Armature Controlled DC Motor
      |
      | $E_a = R_a \cdot I_a + L_a \cdot \frac{di_a}{dt} + K_b \cdot \frac{d\theta}{dt}$
      | $T_{m} = K_{t} \cdot I_{a}$
  Voltage : Inport
  Velocity : Inport  Port=2
  Constant1 : Constant  Value=R
  Gain1 : Gain  Gain=Kb
  Gain2 : Gain  Gain=1/L
  Gain3 : Gain  Gain=Kt
  Integrator : Integrator
  Product : Product
  Subtract : Sum  Inputs=+--
  Tourque : Outport
  wires:
  Voltage/1 -> Subtract/1
  Integrator/1 -> Product/1, Gain3/1  "i"
  Gain3/1 -> Tourque/1
  Gain1/1 -> Subtract/2
  Velocity/1 -> Gain1/1
  Constant1/1 -> Product/2
  Product/1 -> Subtract/3
  Gain2/1 -> Integrator/1  "i_dot"
  Subtract/1 -> Gain2/1

== stateflow chart Conveyer_Belt_System/Sensors1 ==
  state Stationery
    entry:
    Voltage=0;
  state Motion
    entry:
    Voltage=1;
  (default) -> Stationery
  Stationery -> Motion : [Crane==1]
  Motion -> Stationery : [Belt==1]
  data: Crane input; Belt input; Voltage output

== stateflow chart Conveyer_Belt_System/Sensors ==
  state Stationery
    entry:
    Voltage=0;
  state Motion
    entry:
    Voltage=12;
  (default) -> Stationery
  Stationery -> Motion : [Crane==1]
  Motion -> Stationery : [Belt==1]
  data: Crane input; Belt input; Voltage output

== stateflow chart Conveyer_Belt_System/Sensors Logic ==
  note: ?
  state Motor9
    entry:
    V9=12;
  state Motor8
    entry:
    V8=12;
  state Motor7
    entry:
    V7=12;
  state Motor1
    entry:
    V1=12;
  state Stationery
    entry:
    V1=0; V2=0; V3=0; V4=0; V5=0; V6=0;
    V7=0; V8=0; V9=0;
  state Motor2
    entry:
    V2=12;
  state Motor6
    entry:
    V6=12;
  state Motor3
    entry:
    V3=12;
  state Motor5
    entry:
    V5=12;
  state Motor4
    entry:
    V4=12;
  Stationery -> Motor8 [order 8] : [x==8&&y==8]
  Motor8 -> Stationery : [Belt8==1]
  Stationery -> Motor9 [order 9] : [x==9&&y==9]
  Motor9 -> Stationery : [Belt9==1]
  Motor7 -> Stationery : [Belt7==1]
  Stationery -> Motor7 [order 7] : [x==7&&y==7]
  Stationery -> Motor1 [order 1] : [x==1&&y==1]
  Motor1 -> Stationery : [Belt1==1]
  Stationery -> Motor2 [order 2] : [x==2&&y==2]
  Motor6 -> Stationery : [Belt6==1]
  Motor2 -> Stationery : [Belt2==1]
  Stationery -> Motor6 [order 6] : [x==6&&y==6]
  Motor5 -> Stationery : [Belt5==1]
  Stationery -> Motor5 [order 5] : [x==5&&y==5]
  (default) -> Stationery
  Motor4 -> Stationery : [Belt4==1]
  Stationery -> Motor4 [order 4] : [x==4&&y==4]
  Motor3 -> Stationery : [Belt3==1]
  Stationery -> Motor3 [order 3] : [x==3&&y==3]
  data: Belt1 input; Belt2 input; Belt3 input; Belt4 input; Belt5 input; Belt6 input; Belt7 input; Belt8 input; Belt9 input; x input; y input; V1 output; V2 output; V3 output; V4 output; V5 output; V6 output; V7 output; V8 output; V9 output
